simulink model "launch_rail_velocity"  (R2021a)
settings: Solver=VariableStepAuto  StartTime=0.0  StopTime=10.0  RelTol=1e-3
settings Model: Creator=Maderm  LastModifiedBy=Maderm
settings SolverCC: AlgebraicLoopSolver=TrustRegion
settings DebuggingCC: SFMachineParentedDataDiag=warning

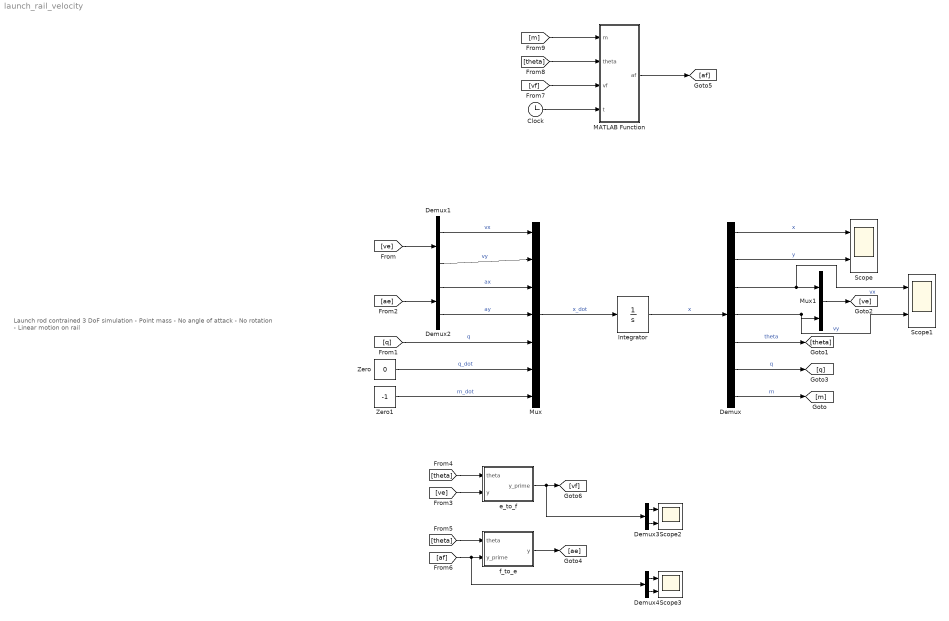
== system launch_rail_velocity ==
  note: Launch rod contrained 3 DoF simulation
      | - Point mass
      | - No angle of attack
      | - No rotation
      | - Linear motion on rail
  Clock : Clock
  Demux : Demux  Outputs=7
  Demux{1..4} (4 alike) : Demux  Outputs=2
  Integrator : Integrator  InitialCondition=[0;0;0;0;85;0;140]
  MATLAB Function : MATLAB Function  TreatAsAtomicUnit=on
  Mux : Mux  Inputs=7
  Mux1 : Mux  Inputs=2
  Scope{,1..3} (4 alike) : Scope  NumInputPorts=2
  Zero : Constant  Value=0  OutDataTypeStr=Inherit: Inherit via back propagation  SampleTime=-1
  Zero1 : Constant  Value=-1  OutDataTypeStr=Inherit: Inherit via back propagation  SampleTime=-1
  e_to_f : MATLAB Function  TreatAsAtomicUnit=on
  f_to_e : MATLAB Function  TreatAsAtomicUnit=on
  wires:
  Mux/1 -> Integrator/1  "x_dot"
  Integrator/1 -> Demux/1  "x"
  Demux1/1 -> Mux/1  "vx"
  Demux1/2 -> Mux/2  "vy"
  Demux2/1 -> Mux/3  "ax"
  Demux2/2 -> Mux/4  "ay"
  [q] -> Mux/5  "q"
  Zero/1 -> Mux/6  "q_dot"
  Zero1/1 -> Mux/7  "m_dot"
  Demux/1 -> Scope/1  "x"
  Demux/2 -> Scope/2  "y"
  Demux/3 -> Scope1/1, Mux1/1  "vx"
  Demux/4 -> Scope1/2, Mux1/2  "vy"
  Demux/5 -> [theta]  "theta"
  Demux/6 -> [q]  "q"
  Demux/7 -> [m]  "m"
  Mux1/1 -> [ve]
  [ve] -> Demux1/1
  [ae] -> Demux2/1
  [ve] -> e_to_f/2(y)
  [theta] -> e_to_f/1(theta)
  f_to_e/1(y) -> [ae]
  [theta] -> f_to_e/1(theta)
  [af] -> Demux4/1, f_to_e/2(y_prime)
  e_to_f/1(y_prime) -> Demux3/1, [vf]
  MATLAB Function/1(af) -> [af]
  Clock/1 -> MATLAB Function/4(t)
  [vf] -> MATLAB Function/3(vf)
  [theta] -> MATLAB Function/2(theta)
  [m] -> MATLAB Function/1(m)
  Demux3/1 -> Scope2/1
  Demux3/2 -> Scope2/2
  Demux4/2 -> Scope3/2
  Demux4/1 -> Scope3/1

== matlab function launch_rail_velocity/f_to_e ==
  data: theta input; y output; y_prime input
function y = fcn(theta,y_prime)

A = [cosd(theta) -sind(theta); sind(theta) cosd(theta)];

y = A'*y_prime;

== matlab function launch_rail_velocity/e_to_f ==
  data: theta input; y_prime output; y input
function y_prime = fcn(theta,y)

A = [cosd(theta) -sind(theta); sind(theta) cosd(theta)];

y_prime = A*y;

== matlab function launch_rail_velocity/MATLAB Function ==
  data: m input; af output; theta input; vf input; t input
function af = fcn(m,theta,vf,t)

g = 9.81;
Cd = 0.5;
Cf = 0.6;
rho = 1.225;
S = pi/4*0.1524^2;

vxf = vf(1);

T = 500*exp(-t/5);

af1 = T/m-g*sind(theta)-sign(vxf)*(g*cosd(theta)*Cf+0.5*rho*vxf^2*S*Cd/m);
af = [af1;0];
